simulink model "enabled_subsystem"  (R2024a)
settings: Solver=FixedStepDiscrete  StartTime=0.0  StopTime=10.0  FixedStep=0.5  RelTol=1e-3
settings Model: Creator=DELL  LastModifiedBy=DELL
settings OptimizationCC: DefaultParameterBehavior=Inlined  EnhancedBackFolding=on  PassReuseOutputArgsAs=Individual arguments  ZeroExternalMemoryAtStartup=off  ZeroInternalMemoryAtStartup=off  OptimizeBlockOrder=speed  DifferentSizesBufferReuse=on  OptimizationCustomize=off  EfficientTunableParamExpr=on
settings DebuggingCC: ParameterTunabilityLossMsg=error
settings SFSimCC: MATLABDynamicMemAlloc=off
settings RTWCC: Description=Embedded Coder  SystemTargetFile=ert.tlc  TemplateMakefile=ert_default_tmf
settings CodeAppCC: ForceParamTrailComments=on  IgnoreCustomStorageClasses=off  OperatorAnnotations=on  SimulinkDataObjDesc=on  SFDataObjDesc=on  InsertBlockDesc=on
settings ERTTargetCC: TargetLangStandard=C99 (ISO)  GenerateSampleERTMain=on  InlinedParameterPlacement=NonHierarchical  ERTCustomFileTemplate=example_file_process.tlc

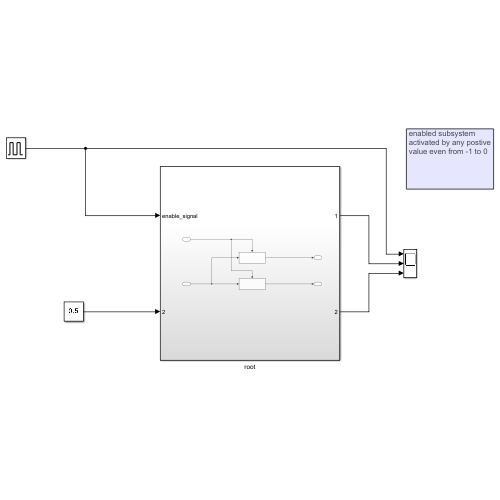
[thumbnail: Simulink's stored preview of the top-level diagram]
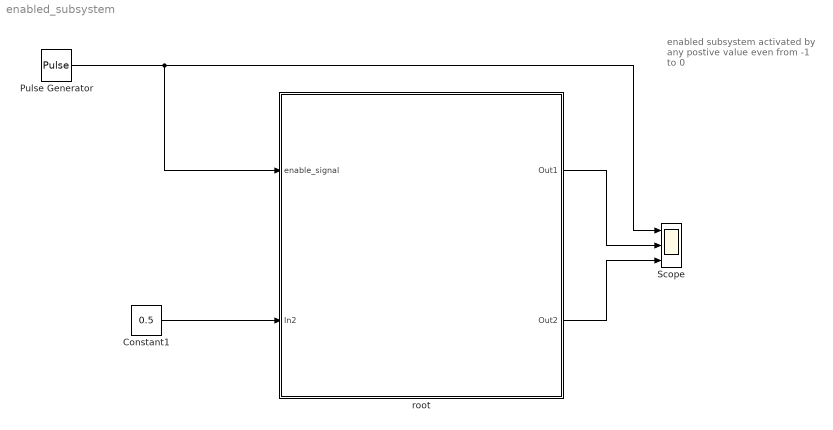
== system enabled_subsystem ==
  note: enabled subsystem
      | activated by any postive
      | value even from -1 to 0
  Constant1 : Constant  Value=0.5
  Pulse Generator : DiscretePulseGenerator  PulseType=Time based  Period=1  PulseWidth=50
  Scope : Scope  NumInputPorts=3
  root : Subsystem
      settings: RTWFcnNameOpts=Use subsystem name
  wires:
  Pulse Generator/1 -> Scope/1, root/1(enable_signal)
  Constant1/1 -> root/2(In2)
  root/1(Out1) -> Scope/2
  root/2(Out2) -> Scope/3

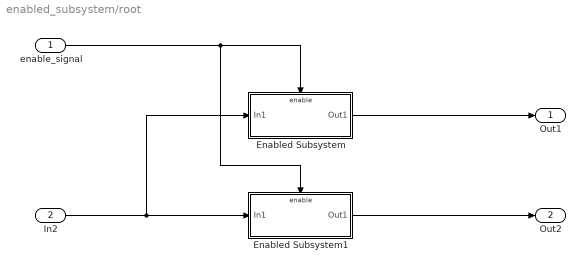
== system enabled_subsystem/root ==
  enable_signal : Inport
  In2 : Inport  Port=2
  Enabled Subsystem : Subsystem  TreatAsAtomicUnit=on
      settings: RTWSystemCode=Nonreusable function
  Enabled Subsystem1 : Subsystem  TreatAsAtomicUnit=on
      settings: RTWSystemCode=Nonreusable function
  Out1 : Outport
  Out2 : Outport  Port=2
  wires:
  In2/1 -> Enabled Subsystem/1(In1), Enabled Subsystem1/1(In1)
  Enabled Subsystem/1(Out1) -> Out1/1
  enable_signal/1 -> Enabled Subsystem/Enable, Enabled Subsystem1/Enable
  Enabled Subsystem1/1(Out1) -> Out2/1

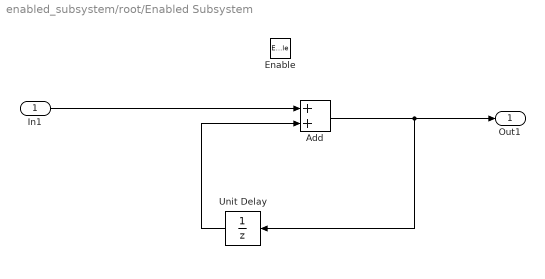
== system enabled_subsystem/root/Enabled Subsystem ==
  In1 : Inport
  Enable : EnablePort
  Add : Sum
  Unit Delay : UnitDelay  SampleTime=-1  HasFrameUpgradeWarning=on
  Out1 : Outport
  wires:
  In1/1 -> Add/1
  Unit Delay/1 -> Add/2
  Add/1 -> Unit Delay/1, Out1/1

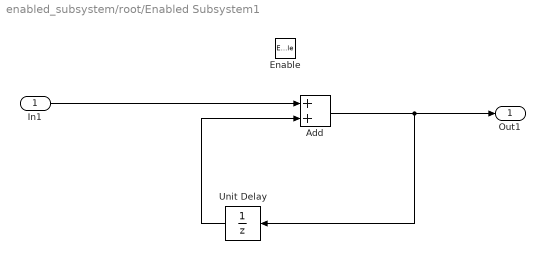
== system enabled_subsystem/root/Enabled Subsystem1 ==
  In1 : Inport
  Enable : EnablePort  StatesWhenEnabling=reset
  Add : Sum
  Unit Delay : UnitDelay  SampleTime=-1  HasFrameUpgradeWarning=on
  Out1 : Outport
  wires:
  Add/1 -> Out1/1, Unit Delay/1
  Unit Delay/1 -> Add/2
  In1/1 -> Add/1
